simulink model "startSunRef"  (R2021a)
settings: Solver=FixedStepAuto  StartTime=0.0  StopTime=10.0  RelTol=1e-3
undefined symbols (not defined in the file): CubeSatTimeStep, IAU, initCond, km, s
libraries: aerolibtransform2 x1, dspmathops x1, aerolibcelestial x1
settings Model: Creator=noraw  LastModifiedBy=noraw

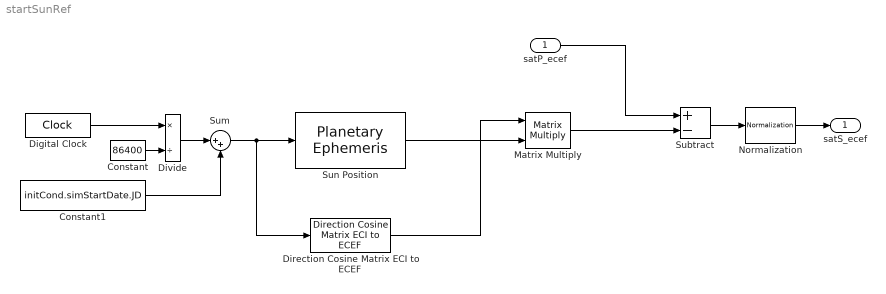
== system startSunRef ==
  satP_ecef : Inport  PortDimensions=3
  Constant : Constant  Value=86400
  Constant1 : Constant  Value=initCond.simStartDate.JD
  Digital Clock : DigitalClock  SampleTime=CubeSatTimeStep
  Direction Cosine Matrix ECI to ECEF : aerolibtransform2/Direction Cosine Matrix ECI to ECEF  red=IAU-2000/2006  year=2019  month=January  day=4  hour=0  min=0  sec=0  deltaT=Day  errorflag=Error  extraparamflag=off
      settings: AttributesFormatString=%<red>  SourceProductBaseCode=AE
  Divide : Product  Inputs=*/
  Matrix Multiply : Product  Multiplication=Matrix(*)
  Normalization : dspmathops/Normalization  NormType=2-norm  Bias=1e-10  NormOver=Each column  Dimension=1  roundingMode=Floor  overflowMode=off  accumDataTypeStr=Inherit: Same as product output  accumLastDataTypeStr=Inherit: Same as product output  outputDataTypeStr=Inherit: Same as product output  outputMin=[]  outputMax=[]  outputLastDataTypeStr=Inherit: Same as product output
  Subtract : Sum  Inputs=+-
  Sum : Sum  Inputs=|++
  Sun Position : aerolibcelestial/Planetary Ephemeris  kmflag=km,km/s  epochflag=Julian date  de=DE421  nCenter=Earth  nTarget=Sun  errorflag=Error  velflag=off
      settings: SourceProductBaseCode=AE
  satS_ecef : Outport
  wires:
  Direction Cosine Matrix ECI to ECEF/1 -> Matrix Multiply/1
  Constant/1 -> Divide/2
  Matrix Multiply/1 -> Subtract/2
  Constant1/1 -> Sum/2
  Sum/1 -> Direction Cosine Matrix ECI to ECEF/1, Sun Position/1
  Digital Clock/1 -> Divide/1
  Divide/1 -> Sum/1
  Sun Position/1 -> Matrix Multiply/2
  satP_ecef/1 -> Subtract/1
  Subtract/1 -> Normalization/1
  Normalization/1 -> satS_ecef/1
